simulink model "LQE"  (R2020a)
settings: Solver=VariableStepAuto  StartTime=0.0  StopTime=20  RelTol=1e-3
values from neighbouring files (symbols this model uses):
  A = stateSpaceModel.A    [System_Control.m]    (also in script2.m)
  B = stateSpaceModel.B    [System_Control.m]    (also in script2.m)
  C = stateSpaceModel.C    [System_Control.m]    (also in script2.m)
  Ts = stateSpaceModel.Ts    [System_Control.m]    (also in script2.m)
undefined symbols (not defined in the file or in its folder): M
settings Model: Creator=Gil  LastModifiedBy=Gil
settings DebuggingCC: ArithmeticOperatorsInVariantConditions=warning
settings SFSimCC: CustomCodeUndefinedFunction=UseInterfaceOnly

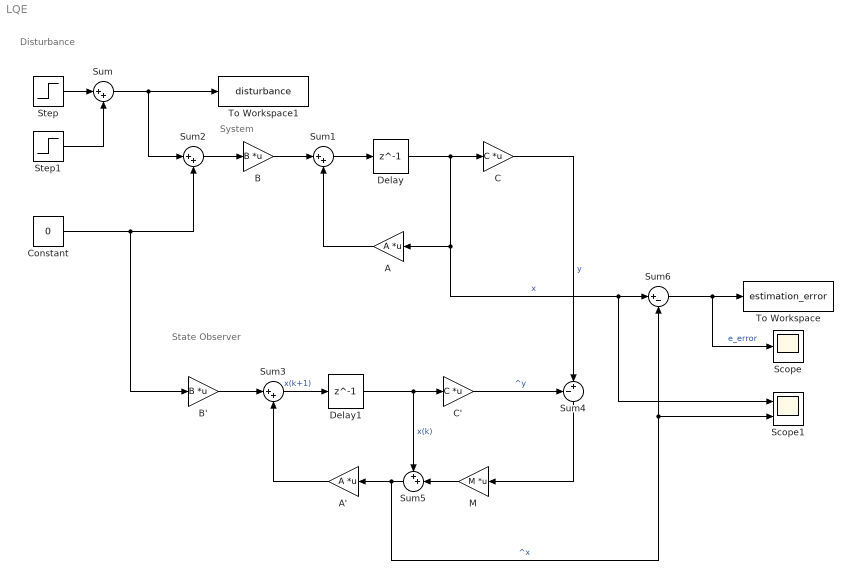
== system LQE ==
  note: Disturbance
  note: System
  note: State Observer
  "A " : Gain  Gain=A  Multiplication=Matrix(K*u)
  A' : Gain  Gain=A  Multiplication=Matrix(K*u)
  B : Gain  Gain=B  Multiplication=Matrix(K*u)
  B' : Gain  Gain=B  Multiplication=Matrix(K*u)
  C : Gain  Gain=C  Multiplication=Matrix(K*u)
  C' : Gain  Gain=C  Multiplication=Matrix(K*u)
  Constant : Constant  Value=0
  Delay : Delay  DelayLength=1  InitialCondition=0  SampleTime=Ts
  Delay1 : Delay  DelayLength=1  InitialCondition=0  SampleTime=Ts
  M : Gain  Gain=M  Multiplication=Matrix(K*u)
  Scope : Scope
  Scope1 : Scope  NumInputPorts=2
  Step : Step  Time=2  Before=-1  SampleTime=Ts
  Step1 : Step  Time=4  Before=1  After=-1  SampleTime=Ts
  Sum{,1..3} (4 alike) : Sum  Inputs=|++
  Sum4 : Sum  Inputs=-+|
  Sum5 : Sum  Inputs=++|
  Sum6 : Sum  Inputs=|+-
  To Workspace : ToWorkspace  VariableName=estimation_error  SaveFormat=Structure With Time  SampleTime=Ts
  To Workspace1 : ToWorkspace  VariableName=disturbance  SaveFormat=Structure With Time  SampleTime=Ts
  wires:
  Sum/1 -> Sum2/1, To Workspace1/1
  Sum2/1 -> B/1
  Step/1 -> Sum/1
  Delay/1 -> Scope1/1, Sum6/1, "A "/1, C/1  "x"
  B/1 -> Sum1/1
  Sum1/1 -> Delay/1
  Step1/1 -> Sum/2
  "A "/1 -> Sum1/2
  Constant/1 -> B'/1, Sum2/2
  Sum4/1 -> M/1
  Sum3/1 -> Delay1/1  "x(k+1)"
  B'/1 -> Sum3/1
  C'/1 -> Sum4/1  "^y"
  C/1 -> Sum4/2  "y"
  M/1 -> Sum5/2
  Delay1/1 -> Sum5/1, C'/1  "x(k)"
  A'/1 -> Sum3/2
  Sum5/1 -> A'/1, Scope1/2, Sum6/2  "^x"
  Sum6/1 -> Scope/1, To Workspace/1  "e_error"
